simulink model "Practica_2_MSF"  (R2025b)
settings: Solver=VariableStepAuto  StartTime=0.0  StopTime=10.0  RelTol=1e-3
libraries: slpidlib x2
settings DataIOCC: ReturnWorkspaceOutputs=off  TimeSaveName=t
settings DebuggingCC: AlgebraicLoopMsg=none  ArtificialAlgebraicLoopMsg=none  MaxConsecutiveZCsMsg=none

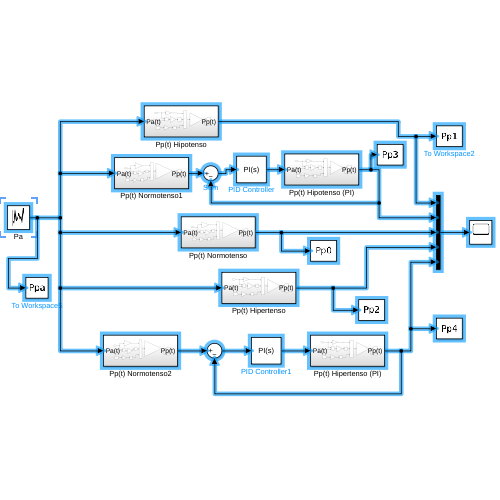
[thumbnail: Simulink's stored preview of the top-level diagram]
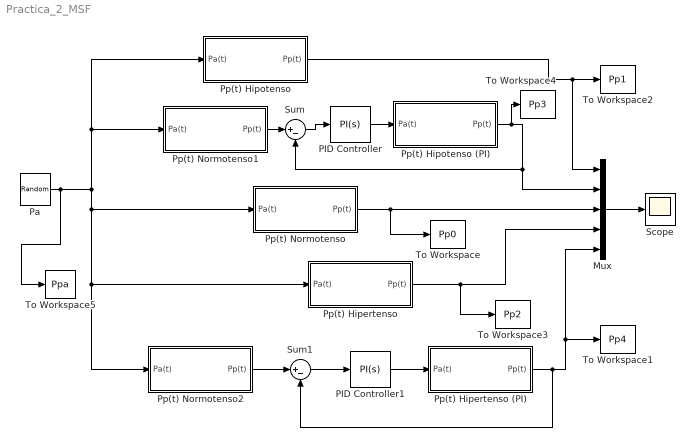
== system Practica_2_MSF ==
  Mux : Mux  Inputs=5
  PID Controller : slpidlib/PID Controller  Controller=PI  Form=Parallel  TimeDomain=Continuous-time  UseExternalTs=off  SampleTime=-1  IntegratorMethod=Forward Euler  FilterMethod=Forward Euler  ControllerParametersSource=internal  P=10  I=3928.62362169833  UseKiTs=off  D=0  UseExternalDerivativeSource=off  N=100  UseFilter=on  TunerSelectOption=Transfer Function Based (PID Tuner App)  InitialConditionSource=internal  InitialConditionForIntegrator=0  InitialConditionForFilter=0  DifferentiatorICPrevScaledInput=0  ExternalReset=none  TrackingMode=off  Kt=1  LimitOutput=off  SatLimitsSource=internal  UpperSaturationLimit=inf  LowerSaturationLimit=-inf  LinearizeAsGain=on  AntiWindupMode=none  Kb=1  LimitIntegrator=off  UpperIntegratorSaturationLimit=inf  LowerIntegratorSaturationLimit=-inf  POutMin=[]  POutMax=[]  IOutMin=[]  IOutMax=[]  DOutMin=[]  DOutMax=[]  NOutMin=[]  NOutMax=[]  SumOutMin=[]  SumOutMax=[]  SaturationOutMin=[]  SaturationOutMax=[]  PParamMin=[]  PParamMax=[]  IParamMin=[]  IParamMax=[]  DParamMin=[]  DParamMax=[]  NParamMin=[]  NParamMax=[]  KbParamMin=[]  KbParamMax=[]  KtParamMin=[]  KtParamMax=[]  KbOutMin=[]  KbOutMax=[]  KtOutMin=[]  KtOutMax=[]  IntegratorOutMin=[]  IntegratorOutMax=[]  FilterOutMin=[]  FilterOutMax=[]  SumI1OutMin=[]  SumI1OutMax=[]  SumI2OutMin=[]  SumI2OutMax=[]  SumI3OutMin=[]  SumI3OutMax=[]  SumI4OutMin=[]  SumI4OutMax=[]  SumDOutMin=[]  SumDOutMax=[]  DifferentiatorOutMin=[]  DifferentiatorOutMax=[]  FilterDiffOutCoefMin=[]  FilterDiffOutCoefMax=[]  ReciprocalOutMin=[]  ReciprocalOutMax=[]  SumDenOutMin=[]  SumDenOutMax=[]  SumNumOutMin=[]  SumNumOutMax=[]  DivideOutMin=[]  DivideOutMax=[]  UdiffTsProdOutMin=[]  UdiffTsProdOutMax=[]  NTsProdOutMin=[]  NTsProdOutMax=[]  UintegralTsProdOutMin=[]  UintegralTsProdOutMax=[]  UngainTsProdOutMin=[]  UngainTsProdOutMax=[]  ClampingZeroOutDataTypeStr=Inherit: Inherit via back propagation  ClampingZeroOutMin=[]  ClampingZeroOutMax=[]  FilterDenConstantOutDataTypeStr=Inherit: Inherit via back propagation  FilterDenConstantOutMin=[]  FilterDenConstantOutMax=[]  PCopyOutDataTypeStr=Inherit: Inherit via back propagation  PCopyOutMin=[]  PCopyOutMax=[]  NCopyOutDataTypeStr=Inherit: Inherit via back propagation  NCopyOutMin=[]  NCopyOutMax=[]  IntegratorContinuousStateAttributes=''  IntegratorStateMustResolveToSignalObject=off  IntegratorRTWStateStorageClass=Auto  FilterContinuousStateAttributes=''  FilterStateMustResolveToSignalObject=off  FilterRTWStateStorageClass=Auto  ParallelPVariant=InternalParameters  IdealPVariant=Disabled  IVariant=InternalParameters  DVariant=Disabled  IntegratorVariant=Continuous  SatVariant=Disabled  AWVariant=Passthrough  PCopyVariant=Disabled  TRVariant=Disabled  FdbkBlocksVariant=Forward  IdealPFdbkVariant=Disabled  SatFdbkVariant=Disabled  DerivativeFilterVariant=Disabled  NVariant=Disabled  NCopyVariant=Disabled_SignalSpec  FilterICVariant=Disabled  IntegratorICVariant=InternalICs  ExternalResetVariant=Disabled  TRSumVariant=Passthrough  SumFdbkVariant=Disabled  SumVariant=Sum_PI  TsampFilterVariant=InternalTs  TsampNgainVariant=Passthrough  TsampIntegralVariant=Disabled_SignalSpec  ExternalSaturationOutDataTypeStr=Inherit: Same as second input  DerivativeSourceVariant=Disabled  PreIntVariant=InternalPreInt
  PID Controller1 : slpidlib/PID Controller  Controller=PI  Form=Parallel  TimeDomain=Continuous-time  UseExternalTs=off  SampleTime=-1  IntegratorMethod=Forward Euler  FilterMethod=Forward Euler  ControllerParametersSource=internal  P=100  I=3937.67589046295  UseKiTs=off  D=0  UseExternalDerivativeSource=off  N=100  UseFilter=on  TunerSelectOption=Transfer Function Based (PID Tuner App)  InitialConditionSource=internal  InitialConditionForIntegrator=0  InitialConditionForFilter=0  DifferentiatorICPrevScaledInput=0  ExternalReset=none  TrackingMode=off  Kt=1  LimitOutput=off  SatLimitsSource=internal  UpperSaturationLimit=inf  LowerSaturationLimit=-inf  LinearizeAsGain=on  AntiWindupMode=none  Kb=1  LimitIntegrator=off  UpperIntegratorSaturationLimit=inf  LowerIntegratorSaturationLimit=-inf  POutMin=[]  POutMax=[]  IOutMin=[]  IOutMax=[]  DOutMin=[]  DOutMax=[]  NOutMin=[]  NOutMax=[]  SumOutMin=[]  SumOutMax=[]  SaturationOutMin=[]  SaturationOutMax=[]  PParamMin=[]  PParamMax=[]  IParamMin=[]  IParamMax=[]  DParamMin=[]  DParamMax=[]  NParamMin=[]  NParamMax=[]  KbParamMin=[]  KbParamMax=[]  KtParamMin=[]  KtParamMax=[]  KbOutMin=[]  KbOutMax=[]  KtOutMin=[]  KtOutMax=[]  IntegratorOutMin=[]  IntegratorOutMax=[]  FilterOutMin=[]  FilterOutMax=[]  SumI1OutMin=[]  SumI1OutMax=[]  SumI2OutMin=[]  SumI2OutMax=[]  SumI3OutMin=[]  SumI3OutMax=[]  SumI4OutMin=[]  SumI4OutMax=[]  SumDOutMin=[]  SumDOutMax=[]  DifferentiatorOutMin=[]  DifferentiatorOutMax=[]  FilterDiffOutCoefMin=[]  FilterDiffOutCoefMax=[]  ReciprocalOutMin=[]  ReciprocalOutMax=[]  SumDenOutMin=[]  SumDenOutMax=[]  SumNumOutMin=[]  SumNumOutMax=[]  DivideOutMin=[]  DivideOutMax=[]  UdiffTsProdOutMin=[]  UdiffTsProdOutMax=[]  NTsProdOutMin=[]  NTsProdOutMax=[]  UintegralTsProdOutMin=[]  UintegralTsProdOutMax=[]  UngainTsProdOutMin=[]  UngainTsProdOutMax=[]  ClampingZeroOutDataTypeStr=Inherit: Inherit via back propagation  ClampingZeroOutMin=[]  ClampingZeroOutMax=[]  FilterDenConstantOutDataTypeStr=Inherit: Inherit via back propagation  FilterDenConstantOutMin=[]  FilterDenConstantOutMax=[]  PCopyOutDataTypeStr=Inherit: Inherit via back propagation  PCopyOutMin=[]  PCopyOutMax=[]  NCopyOutDataTypeStr=Inherit: Inherit via back propagation  NCopyOutMin=[]  NCopyOutMax=[]  IntegratorContinuousStateAttributes=''  IntegratorStateMustResolveToSignalObject=off  IntegratorRTWStateStorageClass=Auto  FilterContinuousStateAttributes=''  FilterStateMustResolveToSignalObject=off  FilterRTWStateStorageClass=Auto  ParallelPVariant=InternalParameters  IdealPVariant=Disabled  IVariant=InternalParameters  DVariant=Disabled  IntegratorVariant=Continuous  SatVariant=Disabled  AWVariant=Passthrough  PCopyVariant=Disabled  TRVariant=Disabled  FdbkBlocksVariant=Forward  IdealPFdbkVariant=Disabled  SatFdbkVariant=Disabled  DerivativeFilterVariant=Disabled  NVariant=Disabled  NCopyVariant=Disabled_SignalSpec  FilterICVariant=Disabled  IntegratorICVariant=InternalICs  ExternalResetVariant=Disabled  TRSumVariant=Passthrough  SumFdbkVariant=Disabled  SumVariant=Sum_PI  TsampFilterVariant=InternalTs  TsampNgainVariant=Passthrough  TsampIntegralVariant=Disabled_SignalSpec  ExternalSaturationOutDataTypeStr=Inherit: Same as second input  DerivativeSourceVariant=Disabled  PreIntVariant=InternalPreInt
  Pa : UniformRandomNumber  Minimum=-0.2  Seed=106  SampleTime=0.5
  Pp(t) Hipertenso : Subsystem
  Pp(t) Hipertenso (PI) : Subsystem
  Pp(t) Hipotenso : Subsystem
  Pp(t) Hipotenso (PI) : Subsystem
  Pp(t) Normotenso : Subsystem
  Pp(t) Normotenso1 : Subsystem
  Pp(t) Normotenso2 : Subsystem
  Scope : Scope
      settings: ActiveDisplayYMinimum=-0.24501251545071479  ActiveDisplayYMaximum=1.107353127959636
  Sum : Sum  Inputs=|+-
  Sum1 : Sum  Inputs=|+-
  To Workspace : ToWorkspace  VariableName=Pp0  SampleTime=-1
  To Workspace1 : ToWorkspace  VariableName=Pp4  SampleTime=-1
  To Workspace2 : ToWorkspace  VariableName=Pp1  SampleTime=-1
  To Workspace3 : ToWorkspace  VariableName=Pp2  SampleTime=-1
  To Workspace4 : ToWorkspace  VariableName=Pp3  SampleTime=-1
  To Workspace5 : ToWorkspace  VariableName=Ppa  SampleTime=-1
  wires:
  Pa/1 -> To Workspace5/1, Pp(t) Normotenso2/1(Pa(t)), Pp(t) Hipertenso/1(Pa(t)), Pp(t) Normotenso/1(Pa(t)), Pp(t) Hipotenso/1(Pa(t)), Pp(t) Normotenso1/1(Pa(t))
  Pp(t) Normotenso/1(Pp(t)) -> To Workspace/1, Mux/3
  Pp(t) Hipotenso/1(Pp(t)) -> To Workspace2/1, Mux/1
  Pp(t) Hipertenso/1(Pp(t)) -> To Workspace3/1, Mux/4
  Mux/1 -> Scope/1
  Pp(t) Normotenso1/1(Pp(t)) -> Sum/1
  Sum/1 -> PID Controller/1
  PID Controller/1 -> Pp(t) Hipotenso (PI)/1(Pa(t))
  Pp(t) Hipotenso (PI)/1(Pp(t)) -> To Workspace4/1, Sum/2, Mux/2
  Pp(t) Normotenso2/1(Pp(t)) -> Sum1/1
  Sum1/1 -> PID Controller1/1
  PID Controller1/1 -> Pp(t) Hipertenso (PI)/1(Pa(t))
  Pp(t) Hipertenso (PI)/1(Pp(t)) -> Sum1/2, To Workspace1/1, Mux/5

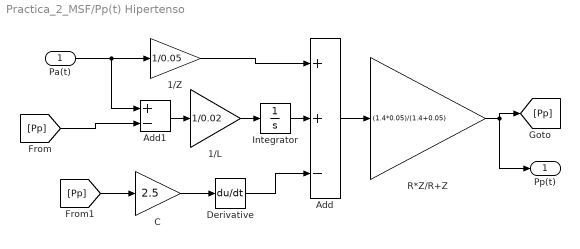
== system Practica_2_MSF/Pp(t) Hipertenso ==
  Pa(t) : Inport
  1/L : Gain  Gain=1/0.02
  1/Z : Gain  Gain=1/0.05
  Add : Sum  Inputs=++-
  Add1 : Sum  Inputs=+-
  C : Gain  Gain=2.5
  Derivative : Derivative
  Integrator : Integrator
  R*Z/R+Z : Gain  Gain=(1.4*0.05)/(1.4+0.05)
  Pp(t) : Outport
  wires:
  Pa(t)/1 -> Add1/1, 1/Z/1
  1/Z/1 -> Add/1
  Add/1 -> R*Z/R+Z/1
  [Pp] -> Add1/2
  R*Z/R+Z/1 -> [Pp], Pp(t)/1
  Add1/1 -> 1/L/1
  1/L/1 -> Integrator/1
  Integrator/1 -> Add/2
  [Pp] -> C/1
  C/1 -> Derivative/1
  Derivative/1 -> Add/3

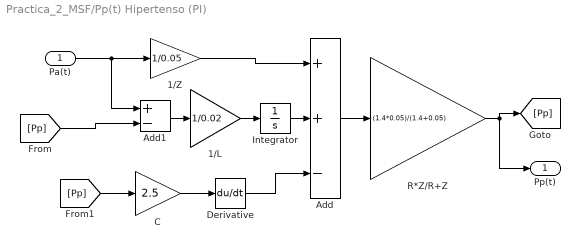
== system Practica_2_MSF/Pp(t) Hipertenso (PI) ==
  Pa(t) : Inport
  1/L : Gain  Gain=1/0.02
  1/Z : Gain  Gain=1/0.05
  Add : Sum  Inputs=++-
  Add1 : Sum  Inputs=+-
  C : Gain  Gain=2.5
  Derivative : Derivative
  Integrator : Integrator
  R*Z/R+Z : Gain  Gain=(1.4*0.05)/(1.4+0.05)
  Pp(t) : Outport
  wires:
  Pa(t)/1 -> Add1/1, 1/Z/1
  1/Z/1 -> Add/1
  Add/1 -> R*Z/R+Z/1
  [Pp] -> Add1/2
  R*Z/R+Z/1 -> [Pp], Pp(t)/1
  Add1/1 -> 1/L/1
  1/L/1 -> Integrator/1
  Integrator/1 -> Add/2
  [Pp] -> C/1
  C/1 -> Derivative/1
  Derivative/1 -> Add/3

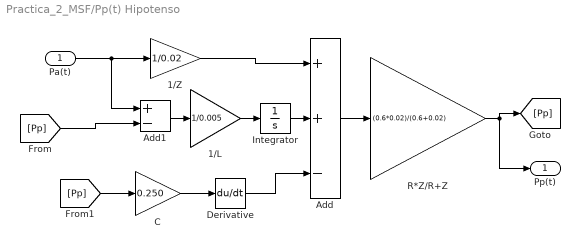
== system Practica_2_MSF/Pp(t) Hipotenso ==
  Pa(t) : Inport
  1/L : Gain  Gain=1/0.005
  1/Z : Gain  Gain=1/0.02
  Add : Sum  Inputs=++-
  Add1 : Sum  Inputs=+-
  C : Gain  Gain=0.250
  Derivative : Derivative
  Integrator : Integrator
  R*Z/R+Z : Gain  Gain=(0.6*0.02)/(0.6+0.02)
  Pp(t) : Outport
  wires:
  Pa(t)/1 -> Add1/1, 1/Z/1
  1/Z/1 -> Add/1
  Add/1 -> R*Z/R+Z/1
  [Pp] -> Add1/2
  R*Z/R+Z/1 -> [Pp], Pp(t)/1
  Add1/1 -> 1/L/1
  1/L/1 -> Integrator/1
  Integrator/1 -> Add/2
  [Pp] -> C/1
  C/1 -> Derivative/1
  Derivative/1 -> Add/3

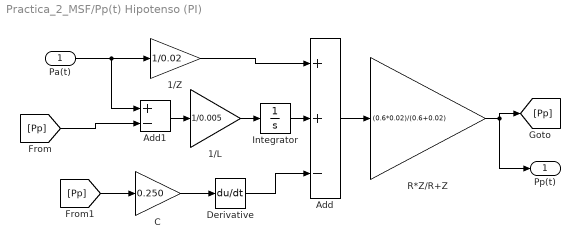
== system Practica_2_MSF/Pp(t) Hipotenso (PI) ==
  Pa(t) : Inport
  1/L : Gain  Gain=1/0.005
  1/Z : Gain  Gain=1/0.02
  Add : Sum  Inputs=++-
  Add1 : Sum  Inputs=+-
  C : Gain  Gain=0.250
  Derivative : Derivative
  Integrator : Integrator
  R*Z/R+Z : Gain  Gain=(0.6*0.02)/(0.6+0.02)
  Pp(t) : Outport
  wires:
  Pa(t)/1 -> Add1/1, 1/Z/1
  1/Z/1 -> Add/1
  Add/1 -> R*Z/R+Z/1
  [Pp] -> Add1/2
  R*Z/R+Z/1 -> [Pp], Pp(t)/1
  Add1/1 -> 1/L/1
  1/L/1 -> Integrator/1
  Integrator/1 -> Add/2
  [Pp] -> C/1
  C/1 -> Derivative/1
  Derivative/1 -> Add/3

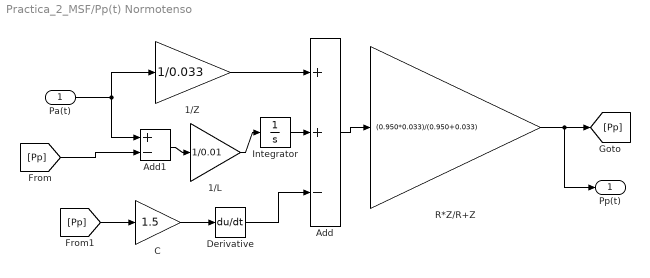
== system Practica_2_MSF/Pp(t) Normotenso ==
  Pa(t) : Inport
  1/L : Gain  Gain=1/0.01
  1/Z : Gain  Gain=1/0.033
  Add : Sum  Inputs=++-
  Add1 : Sum  Inputs=+-
  C : Gain  Gain=1.5
  Derivative : Derivative
  Integrator : Integrator
  R*Z/R+Z : Gain  Gain=(0.950*0.033)/(0.950+0.033)
  Pp(t) : Outport
  wires:
  Pa(t)/1 -> 1/Z/1, Add1/1
  1/Z/1 -> Add/1
  Add/1 -> R*Z/R+Z/1
  [Pp] -> Add1/2
  R*Z/R+Z/1 -> Pp(t)/1, [Pp]
  Add1/1 -> 1/L/1
  1/L/1 -> Integrator/1
  Integrator/1 -> Add/2
  [Pp] -> C/1
  C/1 -> Derivative/1
  Derivative/1 -> Add/3

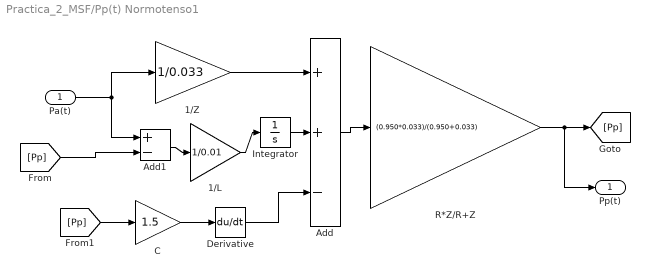
== system Practica_2_MSF/Pp(t) Normotenso1 ==
  Pa(t) : Inport
  1/L : Gain  Gain=1/0.01
  1/Z : Gain  Gain=1/0.033
  Add : Sum  Inputs=++-
  Add1 : Sum  Inputs=+-
  C : Gain  Gain=1.5
  Derivative : Derivative
  Integrator : Integrator
  R*Z/R+Z : Gain  Gain=(0.950*0.033)/(0.950+0.033)
  Pp(t) : Outport
  wires:
  Pa(t)/1 -> 1/Z/1, Add1/1
  1/Z/1 -> Add/1
  Add/1 -> R*Z/R+Z/1
  [Pp] -> Add1/2
  R*Z/R+Z/1 -> Pp(t)/1, [Pp]
  Add1/1 -> 1/L/1
  1/L/1 -> Integrator/1
  Integrator/1 -> Add/2
  [Pp] -> C/1
  C/1 -> Derivative/1
  Derivative/1 -> Add/3

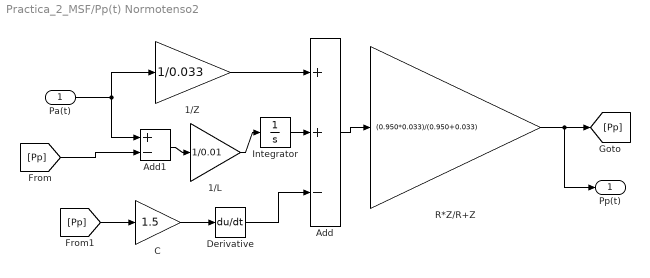
== system Practica_2_MSF/Pp(t) Normotenso2 ==
  Pa(t) : Inport
  1/L : Gain  Gain=1/0.01
  1/Z : Gain  Gain=1/0.033
  Add : Sum  Inputs=++-
  Add1 : Sum  Inputs=+-
  C : Gain  Gain=1.5
  Derivative : Derivative
  Integrator : Integrator
  R*Z/R+Z : Gain  Gain=(0.950*0.033)/(0.950+0.033)
  Pp(t) : Outport
  wires:
  Pa(t)/1 -> 1/Z/1, Add1/1
  1/Z/1 -> Add/1
  Add/1 -> R*Z/R+Z/1
  [Pp] -> Add1/2
  R*Z/R+Z/1 -> Pp(t)/1, [Pp]
  Add1/1 -> 1/L/1
  1/L/1 -> Integrator/1
  Integrator/1 -> Add/2
  [Pp] -> C/1
  C/1 -> Derivative/1
  Derivative/1 -> Add/3
